simulink model "Complete_BTP"  (R2022b)
settings: Solver=VariableStepAuto  StartTime=0.0  StopTime=0.5  RelTol=1e-3
undefined symbols (not defined in the file): Acid, Lead
libraries: spsSeriesRLCBranchLib x7, spsCurrentMeasurementLib x3, simulink x3, spsVoltageMeasurementLib x3, spsDiodeLib x2, spsMosfetLib x2, spsBatteryLib x1, slpidlib x1, spsPVArrayLib x1, spsPWMGeneratorDCDCLib x1, spsParallelRLCBranchLib x1, spspowerguiLib x1
settings Model: Creator=bolt  LastModifiedBy=jishn
settings SolverCC: AlgebraicLoopSolver=TrustRegion
settings DebuggingCC: UnconnectedInputMsg=warning  UnconnectedOutputMsg=warning  UnconnectedLineMsg=warning  SFMachineParentedDataDiag=warning
settings ModelReferenceCC: EnableRefExpFcnMdlSchedulingChecks=on

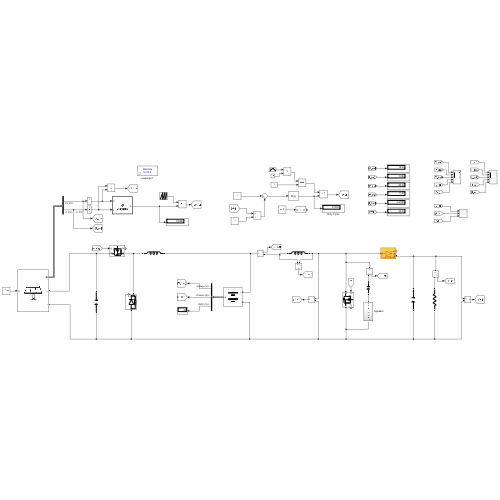
[thumbnail: Simulink's stored preview of the top-level diagram]
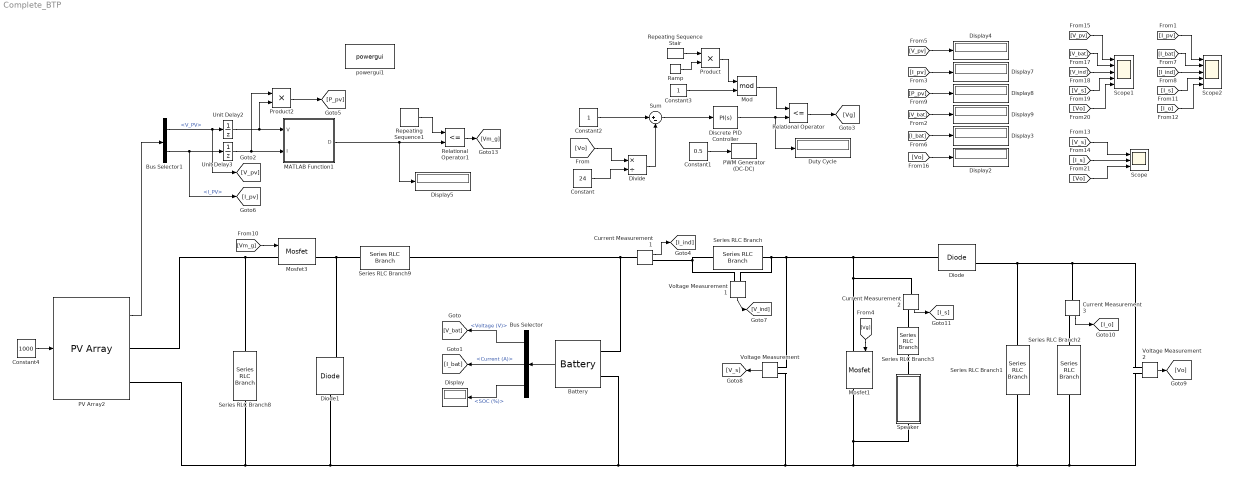
== system Complete_BTP ==
  Battery : spsBatteryLib/Battery  BatType=Lead-Acid  ShowTempParam=off  ThermalPreset=no  ShowAgeParam=off  NomV=12  NomQ=5.4  SOC=50  Batt_Tr=1  PresetModel=on  MaxQ=5.625  MinV=9  FullV=13.0658  Dis_rate=1.08  R=0.022222  Normal_OP=1.6755  expZone="[12.2171        0.018]"  current=[6.5 13 32.5]  Units=Time  Tci=20  NomT=20  T2=-30  MaxQ2=4.8  FullV2=7.1  Normal_OP2=5.655  expZone2="[6.58           1]"  Rca=0.6  ti=2000  Dp=0  Neq0=0  Tsim=1e6  Ta1=25  Qeol=5.4*0.9  Reol=0.013333*1.2  Char_age=[2.3478, 3]  Dis_age=[2.3478, 10]  N1=1500  N2=10500  N3=1000  N4=1400  Ta2=45  N5=950
  Bus Selector : BusSelector  OutputSignals=Voltage (V),Current (A),SOC (%)
  Bus Selector1 : BusSelector  OutputSignals=V_PV,I_PV
  Constant : Constant  Value=24
  Constant1 : Constant  Value=0.5
  Constant2 : Constant
  Constant3 : Constant  SampleTime=1e-6
  Constant4 : Constant  Value=1000
  Current Measurement1 : spsCurrentMeasurementLib/Current Measurement  PhasorSimulation=off  OutputType=Complex  PSBequivalent=0
  Current Measurement2 : spsCurrentMeasurementLib/Current Measurement  PhasorSimulation=off  OutputType=Complex  PSBequivalent=0
  Current Measurement3 : spsCurrentMeasurementLib/Current Measurement  PhasorSimulation=off  OutputType=Complex  PSBequivalent=0
  Diode : spsDiodeLib/Diode  Ron=0.001  Lon=0  Vf=0.8  IC=0  UseSnubber=0  Rs=500  Cs=250e-9  Measurements=on
  Diode1 : spsDiodeLib/Diode  Ron=0.001  Lon=0  Vf=0.8  IC=0  UseSnubber=0  Rs=500  Cs=250e-9  Measurements=on
  Discrete PID Controller : slpidlib/PID Controller  Controller=PI  Form=Parallel  TimeDomain=Continuous-time  UseExternalTs=off  SampleTime=-1  IntegratorMethod=Forward Euler  FilterMethod=Forward Euler  ControllerParametersSource=internal  P=0.1  I=100  UseKiTs=off  D=0  N=100  UseFilter=on  TunerSelectOption=Transfer Function Based (PID Tuner App)  InitialConditionSource=internal  InitialConditionForIntegrator=0  InitialConditionForFilter=0  DifferentiatorICPrevScaledInput=0  ExternalReset=none  TrackingMode=off  Kt=1  LimitOutput=off  SatLimitsSource=internal  UpperSaturationLimit=0.99  LowerSaturationLimit=0.1  LinearizeAsGain=off  AntiWindupMode=none  Kb=1  LimitIntegrator=off  UpperIntegratorSaturationLimit=inf  LowerIntegratorSaturationLimit=-inf  POutMin=[]  POutMax=[]  IOutMin=[]  IOutMax=[]  DOutMin=[]  DOutMax=[]  NOutMin=[]  NOutMax=[]  SumOutMin=[]  SumOutMax=[]  SaturationOutMin=[]  SaturationOutMax=[]  PParamMin=[]  PParamMax=[]  IParamMin=[]  IParamMax=[]  DParamMin=[]  DParamMax=[]  NParamMin=[]  NParamMax=[]  KbParamMin=[]  KbParamMax=[]  KtParamMin=[]  KtParamMax=[]  KbOutMin=[]  KbOutMax=[]  KtOutMin=[]  KtOutMax=[]  IntegratorOutMin=[]  IntegratorOutMax=[]  FilterOutMin=[]  FilterOutMax=[]  SumI1OutMin=[]  SumI1OutMax=[]  SumI2OutMin=[]  SumI2OutMax=[]  SumI3OutMin=[]  SumI3OutMax=[]  SumI4OutMin=[]  SumI4OutMax=[]  SumDOutMin=[]  SumDOutMax=[]  DifferentiatorOutMin=[]  DifferentiatorOutMax=[]  FilterDiffOutCoefMin=[]  FilterDiffOutCoefMax=[]  ReciprocalOutMin=[]  ReciprocalOutMax=[]  SumDenOutMin=[]  SumDenOutMax=[]  SumNumOutMin=[]  SumNumOutMax=[]  DivideOutMin=[]  DivideOutMax=[]  UdiffTsProdOutMin=[]  UdiffTsProdOutMax=[]  NTsProdOutMin=[]  NTsProdOutMax=[]  UintegralTsProdOutMin=[]  UintegralTsProdOutMax=[]  UngainTsProdOutMin=[]  UngainTsProdOutMax=[]  ClampingZeroOutDataTypeStr=Inherit: Inherit via back propagation  ClampingZeroOutMin=[]  ClampingZeroOutMax=[]  FilterDenConstantOutDataTypeStr=Inherit: Inherit via back propagation  FilterDenConstantOutMin=[]  FilterDenConstantOutMax=[]  PCopyOutDataTypeStr=Inherit: Inherit via back propagation  PCopyOutMin=[]  PCopyOutMax=[]  NCopyOutDataTypeStr=Inherit: Inherit via back propagation  NCopyOutMin=[]  NCopyOutMax=[]  IntegratorContinuousStateAttributes=''  IntegratorStateMustResolveToSignalObject=off  IntegratorRTWStateStorageClass=Auto  FilterContinuousStateAttributes=''  FilterStateMustResolveToSignalObject=off  FilterRTWStateStorageClass=Auto  ParallelPVariant=InternalParameters  IdealPVariant=Disabled  IVariant=InternalParameters  DVariant=Disabled  IntegratorVariant=Continuous  SatVariant=Disabled  AWVariant=Passthrough  PCopyVariant=Disabled  TRVariant=Disabled  FdbkBlocksVariant=Forward  IdealPFdbkVariant=Disabled  SatFdbkVariant=Disabled  DerivativeFilterVariant=Disabled  NVariant=Disabled  NCopyVariant=Disabled_SignalSpec  FilterICVariant=Disabled  IntegratorICVariant=InternalICs  ExternalResetVariant=Disabled  TRSumVariant=Passthrough  SumFdbkVariant=Disabled  SumVariant=Sum_PI  TsampFilterVariant=InternalTs  TsampNgainVariant=Passthrough  TsampIntegralVariant=Passthrough  ExternalSaturationOutDataTypeStr=Inherit: Same as second input
  Display{,2..5,7..9} (8 alike) : Display
  Divide : Product  Inputs=*/
  Duty Cycle : Display
  MATLAB Function1 : MATLAB Function  TreatAsAtomicUnit=on
  Mod : Math  Operator=mod
  Mosfet1 : spsMosfetLib/Mosfet  Ron=0.1  Lon=0  Rd=0.01  Vfd=0  IC=0  Rs=1e5  Cs=inf  Measurements=on
  Mosfet3 : spsMosfetLib/Mosfet  Ron=0.1  Lon=0  Rd=0.01  Vfd=0  IC=0  Rs=1e5  Cs=inf  Measurements=on
  PV Array2 : spsPVArrayLib/PV Array  Npar=1  Nser=1  PlotType=array @ 1000 W/m2 & specified temperatures  S_vec="[ 1000  500  100 ]"  Temp_C_vec="[ 45 25  ]"  ModuleName=User-defined  PlotWhenSelected=off  Pm=20.405  Ncell=10  Voc=22.5  Isc=1.1  Vm=19.25  Im=1.06  beta_Voc_pc=-0.36099  alpha_Isc_pc=0.102  beta_Voc=-0.081223  alpha_Isc=0.001122  IL=1.1078  I0=4.0943e-11  nI=3.6462  Rsh=6517.6639  Rs=0.37433  RobustModel=on  RobustCellTemperature=25  BAL=off  Tc=1e-6  Tfilter=5e-5
  PWM Generator (DC-DC) : spsPWMGeneratorDCDCLib/PWM Generator (DC-DC)  Fsw=25000  Ts=0
  Product : Product
  Product2 : Product
  Ramp : simulink/Sources/Ramp  slope=1  start=0  InitialOutput=0
  Relational Operator : RelationalOperator  Operator=<=  OutDataTypeStr=boolean  RndMeth=Simplest  InputSameDT=off
  Relational Operator1 : RelationalOperator  Operator=<=  OutDataTypeStr=boolean  RndMeth=Simplest  InputSameDT=off
  Repeating Sequence Stair : simulink/Sources/Repeating Sequence Stair  OutValues="[20e3  24e3 28e3 32e3 36e3 40e3 36e3 32e3 28e3 24e3 20e3].'"  tsamp=0.2  OutMin=[]  OutMax=[]  OutDataTypeStr=double  OutputDataTypeScalingMode=double  OutDataType=fixdt(0,8)  ConRadixGroup=Best Precision: Vector-wise  OutScaling=2^-12
  Repeating Sequence1 : simulink/Sources/Repeating Sequence  rep_seq_t=[0 0.0004]  rep_seq_y=[0 1]
  Scope : Scope  NumInputPorts=3
  Scope1 : Scope  NumInputPorts=5
  Scope2 : Scope  NumInputPorts=5
  Series RLC Branch : spsSeriesRLCBranchLib/Series RLC Branch  LConnTagsString=__new0  RConnTagsString=__new0  BranchType=L  Resistance=1  Inductance=330e-6  SetiL0=off  InitialCurrent=0  Capacitance=1e-6  Setx0=off  InitialVoltage=0  Measurements=None
  Series RLC Branch1 : spsSeriesRLCBranchLib/Series RLC Branch  LConnTagsString=__new0  RConnTagsString=__new0  BranchType=C  Resistance=1  Inductance=181.8181e-6  SetiL0=off  InitialCurrent=0  Capacitance=1000e-6  Setx0=off  InitialVoltage=240  Measurements=None
  Series RLC Branch2 : spsSeriesRLCBranchLib/Series RLC Branch  LConnTagsString=__new0  RConnTagsString=__new0  BranchType=R  Resistance=50  Inductance=1e-3  SetiL0=off  InitialCurrent=0  Capacitance=1e-6  Setx0=off  InitialVoltage=0  Measurements=None
  Series RLC Branch3 : spsSeriesRLCBranchLib/Series RLC Branch  LConnTagsString=__new0  RConnTagsString=__new0  BranchType=C  Resistance=1  Inductance=181.8181e-6  SetiL0=off  InitialCurrent=0  Capacitance=10e-6  Setx0=off  InitialVoltage=240  Measurements=None
  Series RLC Branch8 : spsSeriesRLCBranchLib/Series RLC Branch  LConnTagsString=__new0  RConnTagsString=__new0  BranchType=C  Resistance=1  Inductance=181.8181e-6  SetiL0=off  InitialCurrent=0  Capacitance=1e-3  Setx0=off  InitialVoltage=240  Measurements=None
  Series RLC Branch9 : spsSeriesRLCBranchLib/Series RLC Branch  LConnTagsString=__new0  RConnTagsString=__new0  BranchType=L  Resistance=1  Inductance=470e-6  SetiL0=off  InitialCurrent=0  Capacitance=1e-6  Setx0=off  InitialVoltage=0  Measurements=None
  Speaker : Subsystem
  Sum : Sum  Inputs=|+-
  Unit Delay2 : UnitDelay  SampleTime=1e-5  HasFrameUpgradeWarning=on
  Unit Delay3 : UnitDelay  SampleTime=1e-5  HasFrameUpgradeWarning=on
  Voltage Measurement : spsVoltageMeasurementLib/Voltage Measurement  PhasorSimulation=off  OutputType=Complex  PSBequivalent=0
  Voltage Measurement1 : spsVoltageMeasurementLib/Voltage Measurement  PhasorSimulation=off  OutputType=Complex  PSBequivalent=0
  Voltage Measurement2 : spsVoltageMeasurementLib/Voltage Measurement  PhasorSimulation=off  OutputType=Complex  PSBequivalent=0
  powergui1 : spspowerguiLib/powergui  Priority=1  SimulationMode=Discrete  SampleTime=1e-6  frequency=60  Iterations=50  frequencyindice=0  Pbase=100e6  ErrMax=1e-4  UnitsV=kV  UnitsW=MW  buscounter=0  FunctionMessages=off  echomessages=off  EnableUseOfTLC=off  CurrentSourceSwitches=off  DisableSnubberDevices=off  DisableRonSwitches=off  DisableVfSwitches=off  DisplayEquations=off  AutomaticDiscreteSolvers=off  SolverType=Tustin/Backward Euler (TBE)  Interpol=off  ExternalGateDelay=off  methode=off  Ts=100  x0status=blocks  SPID=on  SwTol=0  HookPort=off  NonlinearTolerance=1e-4  nMaxIteration=100  ContinueOnMaxIteration=off  RestoreLinks=warning  ResistiveCurrentMeasurement=off  Frange=[0:2:500]  Ylog=off  Xlog=on  ShowGrid=off  save=off  variable=ZData  structure=0  ZoomFFT=off  StartTime=0.0  cycles=1  DisplayStyle=1  fundamental=60  FreqAxis=off  MaxFrequency=1000  frequencyindicesteady=1  RmsSteady=1  display=off
  wires:
  Constant1/1 -> PWM Generator (DC-DC)/1
  [Vg] -> Mosfet1/1
  Constant2/1 -> Sum/1
  [Vo] -> Divide/1
  Constant/1 -> Divide/2
  Divide/1 -> Sum/2
  Relational Operator/1 -> [Vg]
  Discrete PID Controller/1 -> Duty Cycle/1, Relational Operator/2
  Mod/1 -> Relational Operator/1
  Sum/1 -> Discrete PID Controller/1
  Voltage Measurement1/1 -> [V_ind]
  Voltage Measurement/1 -> [V_s]
  Voltage Measurement2/1 -> [Vo]
  Repeating Sequence1/1 -> Relational Operator1/1
  Constant4/1 -> PV Array2/1
  Bus Selector1/2 -> Unit Delay3/1, [I_pv]  "<I_PV>"
  [Vm_g] -> Mosfet3/1
  MATLAB Function1/1(D) -> Display5/1, Relational Operator1/2
  Unit Delay3/1 -> Product2/1, MATLAB Function1/2(I)
  Relational Operator1/1 -> [Vm_g]
  Product2/1 -> [P_pv]
  PV Array2/1 -> Bus Selector1/1
  Bus Selector1/1 -> [V_pv], Unit Delay2/1  "<V_PV>"
  Battery/1 -> Bus Selector/1
  Bus Selector/2 -> [I_bat]  "<Current (A)>"
  Bus Selector/1 -> [V_bat]  "<Voltage (V)>"
  Bus Selector/3 -> Display/1  "<SOC (%)>"
  [I_pv] -> Display7/1
  [V_pv] -> Display4/1
  [I_bat] -> Display3/1
  [Vo] -> Display2/1
  [P_pv] -> Display8/1
  [V_bat] -> Display9/1
  Unit Delay2/1 -> MATLAB Function1/1(V), Product2/2
  Constant3/1 -> Mod/2
  Repeating Sequence Stair/1 -> Product/1
  Product/1 -> Mod/1
  Ramp/1 -> Product/2
  Current Measurement1/1 -> [I_ind]
  [V_pv] -> Scope1/1
  [V_bat] -> Scope1/2
  [V_s] -> Scope1/4
  [V_ind] -> Scope1/3
  [Vo] -> Scope1/5
  [I_ind] -> Scope2/3
  [I_s] -> Scope2/4
  [I_o] -> Scope2/5
  [I_bat] -> Scope2/2
  [I_pv] -> Scope2/1
  Current Measurement2/1 -> [I_s]
  Current Measurement3/1 -> [I_o]
  [V_s] -> Scope/1
  [I_s] -> Scope/2
  [Vo] -> Scope/3
  connections:
  Voltage Measurement2/LConn1 -- Current Measurement3/LConn1 -- Diode/RConn1 -- Series RLC Branch1/LConn1
  Series RLC Branch/RConn1 -- Voltage Measurement1/LConn2 -- Voltage Measurement/LConn1 -- Current Measurement2/LConn1 -- Mosfet1/LConn1 -- Diode/LConn1
  Series RLC Branch/LConn1 -- Current Measurement1/RConn1 -- Voltage Measurement1/LConn1
  Mosfet3/RConn1 -- Series RLC Branch9/LConn1 -- Diode1/RConn1
  PV Array2/RConn1 -- Series RLC Branch8/LConn1 -- Mosfet3/LConn1
  Current Measurement3/RConn1 -- Series RLC Branch2/LConn1
  Series RLC Branch8/RConn1 -- PV Array2/RConn2 -- Diode1/LConn1 -- Voltage Measurement/LConn2 -- Mosfet1/RConn1 -- Speaker/RConn1 -- Voltage Measurement2/LConn2 -- Series RLC Branch2/RConn1 -- Series RLC Branch1/RConn1 -- Battery/LConn2
  Battery/LConn1 -- Current Measurement1/LConn1 -- Series RLC Branch9/RConn1
  Current Measurement2/RConn1 -- Series RLC Branch3/LConn1
  Series RLC Branch3/RConn1 -- Speaker/LConn1

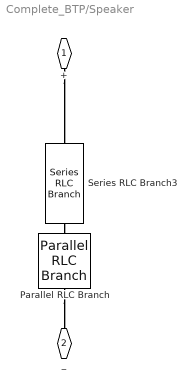
== system Complete_BTP/Speaker ==
  Parallel RLC Branch : spsParallelRLCBranchLib/Parallel RLC Branch  LConnTagsString=a  RConnTagsString=__new0  BranchType=RLC  Resistance=150  Inductance=25e-3  SetiL0=off  InitialCurrent=0  Capacitance=25e-5  Setx0=off  InitialVoltage=0  Measurements=None
  Series RLC Branch3 : spsSeriesRLCBranchLib/Series RLC Branch  LConnTagsString=__new0  RConnTagsString=__new0  BranchType=RL  Resistance=6  Inductance=4e-4  SetiL0=off  InitialCurrent=0  Capacitance=1e-6  Setx0=off  InitialVoltage=0  Measurements=None
  + : PMIOPort  Side=Left
  _ : PMIOPort  Port=2  Side=Right
  connections:
  Series RLC Branch3/RConn1 -- Parallel RLC Branch/LConn1
  +/RConn1 -- Series RLC Branch3/LConn1
  Parallel RLC Branch/RConn1 -- _/RConn1

== matlab function Complete_BTP/MATLAB Function1 ==
  data: V input; D output; I input
function D = DutyRatio(V,I)

Dmax = 0.95;
Dmin = 0;
Dinit =0.95;
deltaD = 0.0001;
persistent Vold Pold Dold;

dataType = 'double';

if isempty(Vold)
    Vold = 0;
    Pold = 0;
    Dold = Dinit;
end

P = V*I;
dV = V-Vold;
dP = P-Pold;

if dP ~=0
    if dP<0
        if dV<0
            D = Dold - deltaD;
        else
            D = Dold + deltaD;
        end
 
    else     
        if dV<0
           D = Dold + deltaD;
        else
           D = Dold - deltaD;
        end
    end

else D = Dold;
end


if D >= Dmax || D <= Dmin
   D = Dold;
end

Dold = D;
Vold = V;
Pold = P;
